simulink model "main_RI_LIEKF_GNSSOutrage"  (R2023a)
settings: Solver=FixedStepAuto  StartTime=0.0  StopTime=220  FixedStep=0.01  RelTol=1e-3
InitFcn:
  | initNavigation0612_AOA;
values from neighbouring files (symbols this model uses):
  CF_enable = 0    [initNavigation.m]
  dt = 0.01    [initNavigation.m]
  dtDelay = -0.03    [initNavigation.m]
  g0 = 9.795    [initNavigation.m]
  gam0_rad = 0/57.3    (= 0)    [initNavigation.m]
  GNSSoutragetime = 90    [initNavigation.m]
  H_sensor_type = 0    [initNavigation.m]
  KF_enable = 1    [initNavigation.m]
  P0 = diag([1*ones(3,1);0.01*ones(3,1);0.1*ones(3,1);0.001*ones(3,1);0.00001*ones(3,1)])    [initNavigation.m]
  P0_RIEKF = diag([1*ones(3,1);0.01*ones(3,1);0.1*ones(3,1);0.001*ones(3,1);0.00001*ones(3,1);      0.01*ones(3,1);[0;2;2]/57.3;[0.1;0.1;0.1]])^2    [initNavigation.m]
  pd0 = 0    [initNavigation.m]
  pe0 = 0    [initNavigation.m]
  phi0_rad = 0/57.3    (= 0)    [initNavigation.m]
  pn0 = 0    [initNavigation.m]
  psi = -178    [initNavigation.m]
  psi0_rad = 0/57.3    (= 0)    [initNavigation.m]
  state_dim = 24    [initNavigation.m]
  Time = 0:0.01:(size(traindata.AttackAngle,1) - 1)*0.01    [NNLiftCoefficientFit.m]
  vd0 = 0    [initNavigation.m]
  ve0 = 0    [initNavigation.m]
  vn0 = 0    [initNavigation.m]
undefined symbols (not defined in the file or in its folder): DiscIntNeverNeededParam, Discrete, INS_CONST, INS_EXPORT, INS_PARAM, magnitude, p, param, pInitialization, sys
libraries: simulink_extras x94, simulink x82, dspstat3 x70, sharedtransform x60, ctrlSharedLib x36, sharedTrackingLibrary x22, matrix_library x15, FMT_Model_Lib x13, deeplib x8, dspsolvers x4, vrlib x4, aerolibconvert2 x1
(part 1 of 28)
settings Model: NumberOfSteps=20  Creator=Ye Xiaoyu  LastModifiedBy=Ye Xiaoyu
settings DataIOCC: SaveFormat=Structure
settings DebuggingCC: ParameterPrecisionLossMsg=none

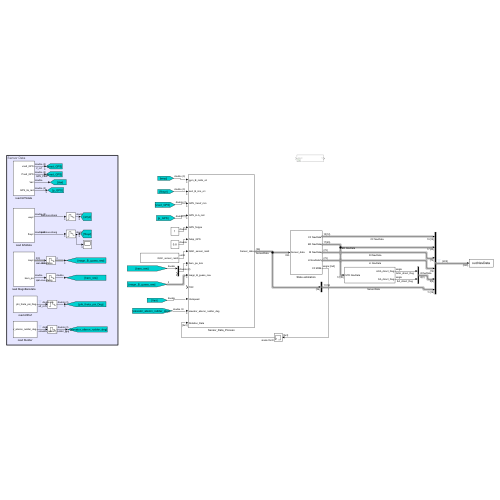
[thumbnail: Simulink's stored preview of the top-level diagram]
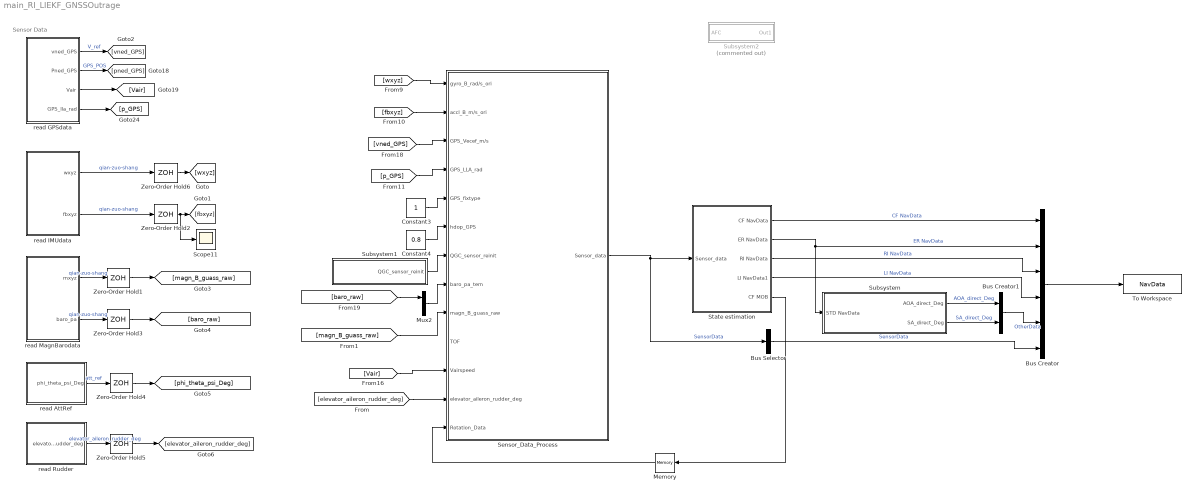
== system main_RI_LIEKF_GNSSOutrage ==
  note: Sensor Data
  Bus Creator : BusCreator  Inputs=6
  Bus Creator1 : BusCreator  Inputs=2
  Bus Selector : BusSelector  OutputSignals=BARO_Data.H_baro_TD,GPS_Data.pos_N_gps,GPS_Data.pos_E_gps,GPS_Data.pos_D_gps,GPS_Data.vn_gps,GPS_Data.ve_gps,GPS_Data.vd_gps,VairspeedData,elevator_aileron_rudder_deg,IMU_Data.gyro_B_rad/s_LPF,IMU_Data.accl_B_m/s2_LPF  OutputAsBus=on
  Constant3 : Constant
  Constant4 : Constant  Value=0.8
  Memory : Memory
  Mux2 : Mux  Inputs=2
  Scope11 : Scope
  Sensor_Data_Process : Subsystem
  State estimation : Subsystem
  Subsystem : Subsystem
  Subsystem1 : Subsystem
  Subsystem2 : Subsystem  Commented=on
  To Workspace : ToWorkspace  VariableName=NavData  SaveFormat=Timeseries  SampleTime=-1
      settings: Save2DSignal=2-D array (concatenate along first dimension)
  Zero-Order Hold{1..6} (6 alike) : ZeroOrderHold  SampleTime=dt
  read AttRef : Subsystem
  read GPSdata : Subsystem
  read IMUdata : Subsystem
  read MagnBarodata : Subsystem
  read Rudder : Subsystem
  wires:
  read GPSdata/2(Pned_GPS) -> [pned_GPS]  "GPS_POS"
  read GPSdata/1(vned_GPS) -> [vned_GPS]  "V_ref"
  read GPSdata/3(Vair) -> [Vair]
  [Vair] -> Sensor_Data_Process/11(Vairspeed)
  [baro_raw] -> Mux2/1
  Zero-Order Hold3/1 -> [baro_raw]
  Zero-Order Hold1/1 -> [magn_B_guass_raw]
  [vned_GPS] -> Sensor_Data_Process/3(GPS_Vecef_m/s)
  read MagnBarodata/2(baro_pa) -> Zero-Order Hold3/1  "qian-zuo-shang"
  Zero-Order Hold6/1 -> [wxyz]
  [p_GPS] -> Sensor_Data_Process/4(GPS_LLA_rad)
  Mux2/1 -> Sensor_Data_Process/8(baro_pa_tem)
  read MagnBarodata/1(mxyz) -> Zero-Order Hold1/1  "qian-zuo-shang"
  Constant4/1 -> Sensor_Data_Process/6(hdop_GPS)
  Constant3/1 -> Sensor_Data_Process/5(GPS_fixtype)
  [magn_B_guass_raw] -> Sensor_Data_Process/9(magn_B_guass_raw)
  [fbxyz] -> Sensor_Data_Process/2(accl_B_m/s_ori)
  Subsystem1/1(QGC_sensor_reinit) -> Sensor_Data_Process/7(QGC_sensor_reinit)
  Zero-Order Hold2/1 -> Scope11/1, [fbxyz]
  Sensor_Data_Process/1(Sensor_data) -> Bus Selector/1, State estimation/1(Sensor_data)  "SensorData"
  read GPSdata/4(GPS_lla_rad) -> [p_GPS]
  read IMUdata/1(wxyz) -> Zero-Order Hold6/1  "qian-zuo-shang"
  [wxyz] -> Sensor_Data_Process/1(gyro_B_rad/s_ori)
  read IMUdata/2(fbxyz) -> Zero-Order Hold2/1  "qian-zuo-shang"
  read AttRef/1(phi_theta_psi_Deg) -> Zero-Order Hold4/1  "att_ref"
  Zero-Order Hold4/1 -> [phi_theta_psi_Deg]
  State estimation/1(CF NavData) -> Bus Creator/1  "CF NavData"
  State estimation/2(ER NavData) -> Subsystem/1(STD NavData), Bus Creator/2  "ER NavData"
  State estimation/3(RI NavData) -> Bus Creator/3  "RI NavData"
  Bus Creator1/1 -> Bus Creator/5  "OtherData"
  Subsystem/1(AOA_direct_Deg) -> Bus Creator1/1  "AOA_direct_Deg"
  Bus Creator/1 -> To Workspace/1
  Subsystem/2(SA_direct_Deg) -> Bus Creator1/2  "SA_direct_Deg"
  Bus Selector/1 -> Bus Creator/6  "SensorData"
  read Rudder/1(elevator_aileron_rudder_deg) -> Zero-Order Hold5/1  "elevator_aileron_rudder_deg"
  Zero-Order Hold5/1 -> [elevator_aileron_rudder_deg]
  [elevator_aileron_rudder_deg] -> Sensor_Data_Process/12(elevator_aileron_rudder_deg)
  State estimation/4(LI NavData1) -> Bus Creator/4  "LI NavData"
  State estimation/5(CF MOB) -> Memory/1
  Memory/1 -> Sensor_Data_Process/13(Rotation_Data)

== system main_RI_LIEKF_GNSSOutrage/Sensor_Data_Process ==
  gyro_B_rad/s_ori : Inport
  accl_B_m/s_ori : Inport  Port=2
  GPS_Vecef_m/s : Inport  Port=3
  GPS_LLA_rad : Inport  Port=4
  GPS_fixtype : Inport  Port=5
  hdop_GPS : Inport  Port=6
  QGC_sensor_reinit : Inport  Port=7
  baro_pa_tem : Inport  Port=8
  magn_B_guass_raw : Inport  Port=9
  TOF : Inport  Port=10
  Vairspeed : Inport  Port=11
  elevator_aileron_rudder_deg : Inport  Port=12
  Rotation_Data : Inport  Port=13
  Bus Creator : BusCreator  Inputs=8
  Data Type Conversion{,1..3,5..6,8..11} (10 alike) : DataTypeConversion  OutDataTypeStr=single  SaturateOnIntegerOverflow=off  RndMeth=Floor
  Data Type Conversion4 : DataTypeConversion  OutDataTypeStr=uint8  SaturateOnIntegerOverflow=off  RndMeth=Floor
  Data Type Conversion7 : DataTypeConversion  OutDataTypeStr=double  SaturateOnIntegerOverflow=off  RndMeth=Floor
  Demux : Demux  Outputs=2
  Digital Clock : DigitalClock  SampleTime=-1
  GPS_Data_Process : Subsystem
  IMU_Data_Process : Subsystem
  Magn_Data_Process1 : Subsystem
  QGC_sensor_reinit1 : InportShadow  Port=7
  QGC_sensor_reinit2 : InportShadow  Port=7
  Subsystem : Subsystem
  TOF_Data_Process : Subsystem
  baro_Data_Process : Subsystem
  Sensor_data : Outport
  wires:
  QGC_sensor_reinit2/1 -> TOF_Data_Process/2(QGC_sensor_reinit)  "QGC_sensor_reinit"
  Data Type Conversion3/1 -> baro_Data_Process/3(baro_tem)
  Demux/2 -> Data Type Conversion3/1
  Data Type Conversion10/1 -> TOF_Data_Process/1(TOF_mm_ori)
  Data Type Conversion5/1 -> baro_Data_Process/1(baro)
  Data Type Conversion9/1 -> GPS_Data_Process/4(hdop_GPS)
  Data Type Conversion4/1 -> GPS_Data_Process/3(GPS_fixtype)
  Data Type Conversion7/1 -> GPS_Data_Process/2(GPS_LLA_rad)
  Data Type Conversion2/1 -> GPS_Data_Process/1(GPS_Vecef_m/s)
  Data Type Conversion1/1 -> IMU_Data_Process/2(accl_B_m/s_ori)
  Data Type Conversion/1 -> IMU_Data_Process/1(gyro_B_rad/s_ori)
  TOF_Data_Process/1(TOF_Data) -> Bus Creator/5
  TOF/1 -> Data Type Conversion10/1
  QGC_sensor_reinit1/1 -> Bus Creator/7  "QGC_sensor_reinit"
  hdop_GPS/1 -> Data Type Conversion9/1
  Bus Creator/1 -> Sensor_data/1
  GPS_fixtype/1 -> Data Type Conversion4/1
  GPS_Vecef_m/s/1 -> Data Type Conversion2/1
  GPS_LLA_rad/1 -> Data Type Conversion7/1
  accl_B_m/s_ori/1 -> Data Type Conversion1/1
  Magn_Data_Process1/1(MAGN_Data) -> Bus Creator/4  "MAGN_Data"
  gyro_B_rad/s_ori/1 -> Data Type Conversion/1
  baro_Data_Process/1(BARO_Data) -> Bus Creator/3  "BARO_Data"
  IMU_Data_Process/1(IMU_Data) -> Bus Creator/1  "IMU_Data"
  GPS_Data_Process/1(GPS_Data) -> Magn_Data_Process1/4(GPS), Bus Creator/2  "GPS_Data"
  QGC_sensor_reinit/1 -> GPS_Data_Process/5(QGC_sensor_reinit), baro_Data_Process/2(QGC_sensor_reinit)  "QGC_sensor_reinit"
  baro_pa_tem/1 -> Demux/1
  Demux/1 -> Data Type Conversion5/1
  Vairspeed/1 -> Data Type Conversion8/1  "VairspeedData"
  Data Type Conversion8/1 -> Subsystem/1(Vairspeed)
  Subsystem/1(VairspeedData) -> Bus Creator/6
  elevator_aileron_rudder_deg/1 -> Data Type Conversion11/1  "elevator_aileron_rudder_deg"
  Data Type Conversion11/1 -> Bus Creator/8  "elevator_aileron_rudder_deg"
  magn_B_guass_raw/1 -> Data Type Conversion6/1
  Data Type Conversion6/1 -> Magn_Data_Process1/1(magn_B_guass_ori)
  Digital Clock/1 -> Magn_Data_Process1/2(magn_B_timestep)
  Rotation_Data/1 -> Magn_Data_Process1/3(Rotation_Data)

== system main_RI_LIEKF_GNSSOutrage/State estimation ==
  Sensor_data : Inport
  0609bk : Subsystem  Commented=on
  15dim KF1 : Subsystem  Commented=on
  Bus Selector : BusSelector  OutputSignals=M_OB
  Bus_Constructor : Subsystem
  Bus_Constructor1 : Subsystem
  Bus_Constructor2 : Subsystem
  Bus_Constructor3 : Subsystem
  Constant : Constant  Value=CF_enable
  Constant1 : Constant  Value=KF_enable
  ER EKF : Subsystem
  LI EKF2 : Subsystem  Commented=on
  RI EKF_AOA_LSTM : Subsystem
  RI EKF_AOA_direct : Subsystem
  RI EKF_AOA_ref : Subsystem
  RI UKF : Subsystem  Commented=on
  bak1 : Subsystem  Commented=on
  distribute CF : Subsystem
  CF NavData : Outport
  ER NavData : Outport  Port=2
  RI NavData : Outport  Port=3
  LI NavData1 : Outport  Port=4
  CF MOB : Outport  Port=5
  wires:
  Sensor_data/1 -> ER EKF/1(Sensor_data), RI EKF_AOA_direct/1(Sensor_data), RI EKF_AOA_ref/1(Sensor_data), RI EKF_AOA_LSTM/1(Sensor_data), RI UKF/1(Sensor_data), distribute CF/1(Sensor_data)
  distribute CF/2(TranslationData) -> Bus_Constructor/2(TranlationData)
  ER EKF/1(RotationData) -> Bus_Constructor1/1(RotationData)
  ER EKF/2(TranslationData) -> Bus_Constructor1/2(TranlationData)
  ER EKF/3(INSbiasData) -> Bus_Constructor1/3(INSbiasData)
  ER EKF/4(EKFstate) -> Bus_Constructor1/4(EKFstate)
  RI EKF_AOA_LSTM/1(RotationData) -> Bus_Constructor2/1(RotationData)
  RI EKF_AOA_LSTM/2(TranslationData) -> Bus_Constructor2/2(TranlationData)
  RI EKF_AOA_LSTM/3(INSbiasData) -> Bus_Constructor2/3(INSbiasData)
  RI EKF_AOA_LSTM/4(EKF_state) -> Bus_Constructor2/4(EKFstate)
  Bus_Constructor/1(CF NavData) -> CF NavData/1
  Bus_Constructor1/1(ER EKFNav_out) -> ER NavData/1
  Bus_Constructor2/1(RI EKFNav_out) -> RI NavData/1
  RI EKF_AOA_LSTM/5(AOA/SA/Wind) -> Bus_Constructor2/5(AOA/SA/Wind)
  RI EKF_AOA_LSTM/6(GNSS enable flag) -> Bus_Constructor2/6(GNSS enable flag)
  RI EKF_AOA_direct/1(RotationData) -> Bus_Constructor3/1(RotationData)
  RI EKF_AOA_direct/2(TranslationData) -> Bus_Constructor3/2(TranlationData)
  RI EKF_AOA_direct/3(INSbiasData) -> Bus_Constructor3/3(INSbiasData)
  RI EKF_AOA_direct/4(EKF_state) -> Bus_Constructor3/4(EKFstate)
  RI EKF_AOA_direct/5(AOA/SA/Wind) -> Bus_Constructor3/5(AOA/SA/Wind)
  RI EKF_AOA_direct/6(GNSS enable flag) -> Bus_Constructor3/6(GNSS enable flag)
  Bus_Constructor3/1(RI EKFNav_out) -> LI NavData1/1
  distribute CF/1(RotationData) -> Bus Selector/1, Bus_Constructor/1(RotationData)
  Bus Selector/1 -> CF MOB/1  "<M_OB>"

== system main_RI_LIEKF_GNSSOutrage/Subsystem ==
  STD NavData : Inport
  Bus Selector : BusSelector  OutputSignals=RotationData.theta_rad,TranlationData.vn_m/s,TranlationData.ve_m/s,TranlationData.vd_m/s,RotationData.psi_rad
  Constant : Constant  Value=0
  Data Type Conversion : DataTypeConversion  OutDataTypeStr=single  SaturateOnIntegerOverflow=off  RndMeth=Floor
  Data Type Conversion1 : DataTypeConversion  OutDataTypeStr=single  SaturateOnIntegerOverflow=off  RndMeth=Floor
  MATLAB Function : MATLAB Function  TreatAsAtomicUnit=on
  Mux : Mux  Inputs=3
  Subsystem1 : Subsystem
  Subsystem3 : Subsystem
  Switch : Switch  Threshold=1  SaturateOnIntegerOverflow=off  InputSameDT=off
  Switch1 : Switch  Threshold=1  SaturateOnIntegerOverflow=off  InputSameDT=off
  AOA_direct_Deg : Outport
  SA_direct_Deg : Outport  Port=2
  wires:
  Bus Selector/2 -> Mux/1  "<vn_m/s>"
  Bus Selector/3 -> Mux/2  "<ve_m/s>"
  STD NavData/1 -> Bus Selector/1
  Bus Selector/4 -> Mux/3  "<vd_m/s>"
  Bus Selector/1 -> Subsystem3/1(RIEKF_att_Deg)  "<theta_rad>"
  Subsystem3/1(AOA_direct_Deg) -> Switch/1
  Mux/1 -> Subsystem1/1(vel_NED), Subsystem3/2(vel_NED)
  Data Type Conversion/1 -> AOA_direct_Deg/1
  Bus Selector/5 -> Subsystem3/3(psi_Deg)  "<psi_rad>"
  Constant/1 -> Switch1/3, Switch/3
  Subsystem1/1(AOA_Estimation_flag) -> Switch1/2, Switch/2, Subsystem3/Enable
  Switch/1 -> Data Type Conversion/1  "INSstate_Rab"
  Subsystem3/2(SA_direct_Deg) -> MATLAB Function/1(dpsi)
  Data Type Conversion1/1 -> SA_direct_Deg/1
  Switch1/1 -> Data Type Conversion1/1  "INSstate_Rab"
  MATLAB Function/1(y) -> Switch1/1

== system main_RI_LIEKF_GNSSOutrage/Subsystem1 ==
  Compare To Constant : simulink/Logic and Bit Operations/Compare To Constant  relop=<=  const=2.1  OutDataTypeStr=boolean
  Compare To Constant1 : simulink/Logic and Bit Operations/Compare To Constant  relop=>=  const=2  OutDataTypeStr=boolean
  Constant5 : Constant  OutDataTypeStr=uint8
  Constant8 : Constant  Value=0  OutDataTypeStr=uint8
  Digital Clock : DigitalClock  SampleTime=dt
  Logical Operator1 : Logic  AllPortsSameDT=off  OutDataTypeStr=boolean
  Switch3 : Switch  Criteria=u2 > Threshold  SaturateOnIntegerOverflow=off  InputSameDT=off
  QGC_sensor_reinit : Outport
  wires:
  Digital Clock/1 -> Compare To Constant1/1, Compare To Constant/1
  Logical Operator1/1 -> Switch3/2
  Constant5/1 -> Switch3/1
  Compare To Constant1/1 -> Logical Operator1/1
  Compare To Constant/1 -> Logical Operator1/2
  Constant8/1 -> Switch3/3
  Switch3/1 -> QGC_sensor_reinit/1

== system main_RI_LIEKF_GNSSOutrage/Subsystem2 ==
  AFC : Inport
  Data Type Conversion18 : DataTypeConversion  OutDataTypeStr=single  SaturateOnIntegerOverflow=off  RndMeth=Floor
  Demux : Demux  Outputs=3
  MATLAB Function1 : MATLAB Function  TreatAsAtomicUnit=on
  Mux2 : Mux  Inputs=2
  Mux29 : Mux  Inputs=2
  Out1 : Outport
  wires:
  Mux2/1 -> Mux29/1
  Data Type Conversion18/1 -> Mux29/2  "AFC"
  Demux/2 -> Mux2/2
  Demux/1 -> Mux2/1
  Demux/3 -> MATLAB Function1/1(x)
  Mux29/1 -> Out1/1
  MATLAB Function1/1(angleHeadingAB0to360) -> Data Type Conversion18/1
  AFC/1 -> Demux/1

== system main_RI_LIEKF_GNSSOutrage/read AttRef ==
  From Workspace : FromWorkspace  VariableName=[All.t',All.thetaL]
  From Workspace1 : FromWorkspace  VariableName=[All.t',All.phiL]
  From Workspace2 : FromWorkspace  VariableName=[All.t',All.psiL]
  Mux3 : Mux  Inputs=3
  phi_theta_psi_Deg : Outport
  wires:
  Mux3/1 -> phi_theta_psi_Deg/1
  From Workspace/1 -> Mux3/2
  From Workspace1/1 -> Mux3/1
  From Workspace2/1 -> Mux3/3

== system main_RI_LIEKF_GNSSOutrage/read GPSdata ==
  Add1 : Sum
  Add2 : Sum
  Constant1 : Constant  Value=1.7
  Constant2 : Constant  Value=0.5311
  Degrees to Radians : simulink_extras/Transformations/Degrees to Radians
  Degrees to Radians1 : simulink_extras/Transformations/Degrees to Radians
  From Workspace : FromWorkspace  VariableName=[All.t',All.ve]
  From Workspace1 : FromWorkspace  VariableName=[All.t',All.vn]
  From Workspace2 : FromWorkspace  VariableName=[All.t',All.mhdot]
  From Workspace3 : FromWorkspace  VariableName=[All.t',All.Yeast]
  From Workspace4 : FromWorkspace  VariableName=[All.t',All.Xnorth]
  From Workspace5 : FromWorkspace  VariableName=[All.t',All.mh]
  From Workspace6 : FromWorkspace  VariableName=[All.t',All.Vc]
  From Workspace7 : FromWorkspace  VariableName=[All.t',All.lat]
  From Workspace8 : FromWorkspace  VariableName=[All.t',All.lon]
  From Workspace9 : FromWorkspace  VariableName=[All.t',All.mh]
  Gain : Gain  Gain=1/3.6
  Gain1 : Gain  Gain=-1
  Gain2 : Gain  Gain=-1
  Gain3 : Gain  Gain=1.0626
  Mux : Mux  Inputs=3
  Mux1 : Mux  Inputs=3
  Mux2 : Mux  Inputs=3
  Scope{,1..2,4} (4 alike) : Scope
  vned_GPS : Outport
  Pned_GPS : Outport  Port=2
  Vair : Outport  Port=3
  GPS_lla_rad : Outport  Port=4
  wires:
  From Workspace2/1 -> Gain1/1
  From Workspace5/1 -> Gain2/1
  From Workspace/1 -> Mux/2  "ve"
  From Workspace1/1 -> Mux/1  "vn"
  From Workspace6/1 -> Gain/1
  From Workspace4/1 -> Mux1/1
  From Workspace3/1 -> Mux1/2
  Gain1/1 -> Mux/3
  Gain2/1 -> Mux1/3
  From Workspace9/1 -> Mux2/3  "altitude"
  Mux2/1 -> Scope/1, GPS_lla_rad/1
  From Workspace8/1 -> Degrees to Radians1/1  "lon"
  From Workspace7/1 -> Degrees to Radians/1  "lat"
  Degrees to Radians/1 -> Mux2/1
  Degrees to Radians1/1 -> Mux2/2
  Mux1/1 -> Pned_GPS/1, Scope1/1
  Mux/1 -> vned_GPS/1, Scope2/1
  Add1/1 -> ?
  Constant1/1 -> Add1/2
  ? -> Scope4/1
  ? -> Add1/1
  Gain/1 -> Gain3/1
  Gain3/1 -> Add2/1
  Constant2/1 -> Add2/2
  Add2/1 -> Vair/1

== system main_RI_LIEKF_GNSSOutrage/read IMUdata ==
  Bus Creator : BusCreator  Inputs=3
  Bus Creator1 : BusCreator  Inputs=3
  Degrees to Radians : simulink_extras/Transformations/Degrees to Radians
  From Workspace : FromWorkspace  VariableName=[All.t',All.q]
  From Workspace1 : FromWorkspace  VariableName=[All.t',All.p]
  From Workspace2 : FromWorkspace  VariableName=[All.t',All.r]
  From Workspace3 : FromWorkspace  VariableName=[All.t',All.Nx]
  From Workspace4 : FromWorkspace  VariableName=[All.t',All.Ny]
  From Workspace5 : FromWorkspace  VariableName=[All.t',All.Nz]
  Gain1 : Gain  Gain=-1
  Gain2 : Gain  Gain=9.81
  Scope : Scope
  Scope1 : Scope
  Scope2 : Scope
  wxyz : Outport
  fbxyz : Outport  Port=2
  wires:
  Bus Creator1/1 -> Scope1/1, Gain2/1
  Bus Creator/1 -> Degrees to Radians/1, Scope/1
  Gain2/1 -> fbxyz/1
  From Workspace2/1 -> Bus Creator/3
  From Workspace5/1 -> Gain1/1
  From Workspace3/1 -> Bus Creator1/1
  From Workspace4/1 -> Bus Creator1/2
  Gain1/1 -> Bus Creator1/3
  From Workspace1/1 -> Bus Creator/1
  From Workspace/1 -> Bus Creator/2
  Degrees to Radians/1 -> Scope2/1, wxyz/1

== system main_RI_LIEKF_GNSSOutrage/read MagnBarodata ==
  Bus Creator : BusCreator  Inputs=3
  From Workspace1 : FromWorkspace  VariableName=[All.t',All.mx]
  From Workspace2 : FromWorkspace  VariableName=[All.t',All.my]
  From Workspace3 : FromWorkspace  VariableName=[All.t',All.baro]
  From Workspace6 : FromWorkspace  VariableName=[All.t',All.mz]
  Gain1 : Gain  Gain=-1
  Scope : Scope
  Scope1 : Scope
  mxyz : Outport
  baro_pa : Outport  Port=2
  wires:
  From Workspace2/1 -> Bus Creator/2
  From Workspace1/1 -> Bus Creator/1
  Bus Creator/1 -> mxyz/1, Scope/1
  From Workspace3/1 -> baro_pa/1
  From Workspace6/1 -> Gain1/1
  Gain1/1 -> Bus Creator/3

== system main_RI_LIEKF_GNSSOutrage/read Rudder ==
  From Workspace : FromWorkspace  VariableName=[All.t',All.dacl]
  From Workspace1 : FromWorkspace  VariableName=[All.t',All.decl]
  From Workspace2 : FromWorkspace  VariableName=[All.t',All.drcl]
  Mux3 : Mux  Inputs=3
  elevator_aileron_rudder_deg : Outport
  wires:
  Mux3/1 -> elevator_aileron_rudder_deg/1
  From Workspace/1 -> Mux3/2
  From Workspace1/1 -> Mux3/1
  From Workspace2/1 -> Mux3/3

== system main_RI_LIEKF_GNSSOutrage/Sensor_Data_Process/GPS_Data_Process ==
  note: GPS_fixtype:
      | 0: 定位不可用或无效
      | 1:单点定位
      | 2:伪距差分
      | 4:RTK固定解
  GPS_Vecef_m/s : Inport
  GPS_LLA_rad : Inport  Port=2
  GPS_fixtype : Inport  Port=3
  hdop_GPS : Inport  Port=4
  QGC_sensor_reinit : Inport  Port=5
  Bus Creator : BusCreator  Inputs=13
  Demux : Demux  Outputs=3
  Demux1 : Demux  Outputs=3
  Demux3 : Demux  Outputs=3
  GPS_fixtype1 : InportShadow  Port=3
  LLA2NED : Subsystem
  heading_GPS : Subsystem
  GPS_Data : Outport
  wires:
  hdop_GPS/1 -> Bus Creator/13  "hdop_GPS"
  heading_GPS/2(heading_GPS_valid) -> Bus Creator/11  "heading_GPS_valid"
  heading_GPS/1(heading_GPS_rad) -> Bus Creator/10  "heading_GPS_rad"
  LLA2NED/2(gpsvNEDout) -> Demux/1
  GPS_Vecef_m/s/1 -> LLA2NED/3(GPS_Vecef_m/s)
  Demux1/3 -> Bus Creator/6  "pos_D_gps"
  Demux1/2 -> Bus Creator/5  "pos_E_gps"
  Demux1/1 -> Bus Creator/4  "pos_N_gps"
  QGC_sensor_reinit/1 -> LLA2NED/4(QGC_sensor_reinit)  "QGC_sensor_reinit"
  GPS_fixtype/1 -> Bus Creator/12  "fixtype_gps"
  Demux3/1 -> Bus Creator/1  "lat_gps"
  Demux3/2 -> Bus Creator/2  "lon_gps"
  Demux/2 -> Bus Creator/8  "ve_gps"
  GPS_LLA_rad/1 -> LLA2NED/1(gps_LLA_rad), Demux3/1
  Demux/1 -> Bus Creator/7  "vn_gps"
  Demux/3 -> Bus Creator/9  "vd_gps"
  Demux3/3 -> Bus Creator/3  "H_gps"
  Bus Creator/1 -> GPS_Data/1
  GPS_fixtype1/1 -> LLA2NED/2(GPSfixtype)  "fixtype_gps"
  LLA2NED/1("gpsposNEDout ") -> Demux1/1, heading_GPS/1(Vned)

== system main_RI_LIEKF_GNSSOutrage/Sensor_Data_Process/IMU_Data_Process ==
  gyro_B_rad/s_ori : Inport
  accl_B_m/s_ori : Inport  Port=2
  Bias Eliminate : Subsystem
  Bus Creator : BusCreator  Inputs=2
  accl_preprocessing2 : Subsystem  Commented=on
  gyro_preprocessing2 : Subsystem  Commented=on
  IMU_Data : Outport  PortDimensions=6
  wires:
  gyro_B_rad/s_ori/1 -> Bias Eliminate/1(gyro_B_rad/s_ori)  "gyro_B_rad/s_LPF"
  Bias Eliminate/1(Out1) -> Bus Creator/1  "gyro_B_rad/s_LPF"
  accl_B_m/s_ori/1 -> Bus Creator/2  "accl_B_m/s2_LPF"
  Bus Creator/1 -> IMU_Data/1

== system main_RI_LIEKF_GNSSOutrage/Sensor_Data_Process/Magn_Data_Process1 ==
  magn_B_guass_ori : Inport
  magn_B_timestep : Inport  Port=2
  Rotation_Data : Inport  Port=3
  GPS : Inport  Port=4
  Bus Creator : BusCreator  Inputs=2
  Gauss_to_uT : Gain  Gain=100
  Mag_Data_Process : Subsystem
  Scope : Scope
  Sensor_Valid : Subsystem  mask{mag_min=-30000, mag_max=30000, timeout=1000}
      mask prompts: mag_min "Mag min (gauss)"; mag_max "Mag max (gauss)"; timeout "Timeout (ms)"
  Zero-Order Hold : ZeroOrderHold  SampleTime=-1
  MAGN_Data : Outport
  wires:
  magn_B_guass_ori/1 -> Gauss_to_uT/1, Sensor_Valid/1(mag_B_gauss)
  magn_B_timestep/1 -> Sensor_Valid/2(timestamp_ms)
  Gauss_to_uT/1 -> Mag_Data_Process/1(mag_B_uT)
  Sensor_Valid/1(valid) -> Scope/1, Mag_Data_Process/2(mag_valid)
  Rotation_Data/1 -> Mag_Data_Process/3(DCM_OB)
  GPS/1 -> Mag_Data_Process/4(GPS_Data)
  Bus Creator/1 -> MAGN_Data/1
  Mag_Data_Process/1(mag_normalized_B) -> Zero-Order Hold/1  "mag_norm_B"
  Mag_Data_Process/2(mag_quality) -> Bus Creator/2  "mag_quality"
  Zero-Order Hold/1 -> Bus Creator/1  "mag_norm_B"

== system main_RI_LIEKF_GNSSOutrage/Sensor_Data_Process/Subsystem ==
  Vairspeed : Inport
  Constant : Constant  Value=0  OutDataTypeStr=single
  Mux : Mux  Inputs=3
  TD_baro : Subsystem
  Terminator : Terminator
  VairspeedData : Outport
  wires:
  TD_baro/2(H_baro_TD) -> Mux/1
  Constant/1 -> Mux/3, Mux/2
  Mux/1 -> VairspeedData/1  "VairspeedData"
  Vairspeed/1 -> TD_baro/1(H_baro)
  TD_baro/1(vH_baro_TD) -> Terminator/1  "vH_baro_m/s_TD"

== system main_RI_LIEKF_GNSSOutrage/Sensor_Data_Process/TOF_Data_Process ==
  TOF_mm_ori : Inport
  QGC_sensor_reinit : Inport  Port=2
  Bus Creator1 : BusCreator  Inputs=4
  Data Type Conversion : DataTypeConversion  OutDataTypeStr=uint8  SaturateOnIntegerOverflow=off  RndMeth=Floor
  Data Type Conversion1 : DataTypeConversion  OutDataTypeStr=single  SaturateOnIntegerOverflow=off  RndMeth=Floor
  Demux : Demux  Outputs=3
  Gain : Gain  Gain=0.01
  Scope : Scope  NumInputPorts=2
  Scope1 : Scope  NumInputPorts=2
  Sum : Sum  Inputs=|-+
  TD_baro : Subsystem
  reinit_TOF : Subsystem
  TOF_Data : Outport
  wires:
  Sum/1 -> Data Type Conversion1/1, Scope1/2  "TOF_Dist_m"
  reinit_TOF/1(dataout) -> Sum/1, Scope1/1
  QGC_sensor_reinit/1 -> reinit_TOF/1(QGC_sensor_reinit)
  Data Type Conversion/1 -> Bus Creator1/4  "TOF_sts"
  Gain/1 -> reinit_TOF/2(Data), Sum/2  "TOF_Dist_m"
  TD_baro/1(vH_TOF_TD) -> Bus Creator1/1, Scope/1  "vH_TOF_m/s_TD"
  Bus Creator1/1 -> TOF_Data/1  "TOF_Data"
  Demux/2 -> Bus Creator1/3  "TOF_Inten"
  TOF_mm_ori/1 -> Demux/1
  Demux/1 -> Gain/1
  Demux/3 -> Data Type Conversion/1  "TOF_sts"
  TD_baro/2(H_TOF_TD) -> Scope/2, Bus Creator1/2  "H_TOF_TD"
  Data Type Conversion1/1 -> TD_baro/1(H_TOF)  "补偿姿态前"

== system main_RI_LIEKF_GNSSOutrage/Sensor_Data_Process/baro_Data_Process ==
  baro : Inport
  QGC_sensor_reinit : Inport  Port=2
  baro_tem : Inport  Port=3
  Add : Sum
  Bus Creator : BusCreator  Inputs=2
  Constant : Constant  Value=0  OutDataTypeStr=single
  Constant1 : Constant  Value=-0.2704  OutDataTypeStr=single
  From Workspace : FromWorkspace  Commented=on  VariableName=[All.t',All.Alt_Ps]
  Gain : Gain  Gain=0.01
  Gain1 : Gain  Gain=1.0530
  Pressure2Height : Subsystem
  Scope : Scope
  Scope1 : Scope  Commented=on  NumInputPorts=2
  Sum : Sum  Inputs=|+-
  Sum1 : Sum  Commented=on  Inputs=|+-
  Sum2 : Sum  Inputs=|+-
  Switch : Switch  Criteria=u2 > Threshold  Threshold=31  SaturateOnIntegerOverflow=off  InputSameDT=off
  TD_baro : Subsystem
  TemCompensate1 : Subsystem
  To Workspace : ToWorkspace  VariableName=H_baro_TD  SaveFormat=Timeseries  SampleTime=-1
  reinit_baro0 : Subsystem
  reinit_baro1 : Subsystem  Commented=on
  BARO_Data : Outport  PortDimensions=2
  wires:
  baro_tem/1 -> TemCompensate1/1(baro_tem), Switch/2  "AFCbarotem"
  Add/1 -> TD_baro/1(H_baro)  "AFC4"
  Switch/1 -> Sum2/2
  baro/1 -> Gain/1  "AFC4"
  Constant/1 -> Switch/1
  TemCompensate1/1(bias) -> Switch/3
  Sum2/1 -> Sum/1, reinit_baro0/2(Data)
  TD_baro/2(H_baro_TD) -> Sum2/1  "H_baro_TD"
  Sum/1 -> Scope1/2, Scope/1, To Workspace/1, Bus Creator/2  "H_baro_TD"
  reinit_baro0/1(dataout) -> Sum/2
  QGC_sensor_reinit/1 -> reinit_baro1/1(QGC_sensor_reinit), reinit_baro0/1(QGC_sensor_reinit)
  Bus Creator/1 -> BARO_Data/1
  Gain/1 -> Pressure2Height/1(baro)
  TD_baro/1(vH_baro_TD) -> Bus Creator/1  "vH_baro_m/s_TD"
  From Workspace/1 -> reinit_baro1/2(Data), Sum1/1
  reinit_baro1/1(dataout) -> Sum1/2
  Sum1/1 -> Scope1/1
  Pressure2Height/1(H_baro) -> Gain1/1  "AFC4"
  Gain1/1 -> Add/1  "AFC4"
  Constant1/1 -> Add/2

== system main_RI_LIEKF_GNSSOutrage/State estimation/0609bk ==
  Sensor_data : Inport
  Bus_Constructor : Subsystem
  Data Store Memory : DataStoreMemory  DataStoreName=feedback_flag_18dim  WriteAfterWriteMsg=warning  ShowAdditionalParam=off
  Data Store Memory1 : DataStoreMemory  DataStoreName=GPS_enable  WriteAfterWriteMsg=warning  ShowAdditionalParam=off
  Data Store Read : DataStoreRead  DataStoreName=GPS_enable  IndexOptions=Index vector (dialog)  Indices=1  OutputSizes=1
  Error State Kalman Filter : Subsystem
  INS propogation : Subsystem
  Sensor_data1 : InportShadow
  TranslationData : Outport
  RotationData : Outport  Port=2
  delta_state : Outport  Port=3
  wires:
  Sensor_data1/1 -> Error State Kalman Filter/1(Sensor_data)
  Bus_Constructor/2(RotationData) -> RotationData/1
  Bus_Constructor/1(TranslationData) -> TranslationData/1
  INS propogation/1(INSstate) -> Bus_Constructor/1(INSstate), Error State Kalman Filter/2(INS state)
  Sensor_data/1 -> INS propogation/1(Sensor_data)
  Error State Kalman Filter/1(state) -> INS propogation/2(state)

== system main_RI_LIEKF_GNSSOutrage/State estimation/15dim KF1 ==
  Sensor_data : Inport
  Bus_Constructor : Subsystem
  Data Store Memory : DataStoreMemory  DataStoreName=feedback_flag  WriteAfterWriteMsg=warning  ShowAdditionalParam=off
  Error State Kalman Filter : Subsystem
  INS propogation : Subsystem
  Scope : Scope
  Sensor_data1 : InportShadow
  Subsystem2 : Subsystem  Commented=on
      settings: PortSchema="{\"entries\":[{\"content\":{\"sides\":[{\"content\":{\"connectorIds\":[\"In1\",\"In2\",\"In3\",\"In4\",\"In5\",\"In6\",\"In7\"]},\"type\":\"ConnectorPlacement.EquallySpacedRectSide\",\"uuid\":\"d8a1abfc-3a64-4957-9a04-f862f8438181\"},{\"content\":{\"connectorIds\":[\"Out1\",\"Out2\"],\"side\":\"RIGHT\"},\"type\":\"ConnectorPlacement.EquallySpacedRectSide\",\"uuid\":\"ef8725ce-d750-4a63-8901-4156c775c830\"},{\"content\":{\"connectorIds\":[\"In8\"],\"side\":\"TOP\"},\"type\":\"ConnectorPlacement.EquallySpacedRectSide\",\"uuid\":\"854b71eb-e012-4efc-86b0-6708fad9ae5c\"},{\"content\":{\"connectorIds\":[],\"side\":\"BOTTOM\"},\"type\":\"ConnectorPlacement.EquallySpacedRectSide\",\"uuid\":\"0d7ed0fe-5852-4514-b91b-1c224e1f49d3\"}]},\"type\":\"ConnectorPlacement.EquallySpacedConnector\",\"uuid\":\"3a6989db-34d3-4b77-867e-5841d7913155\"}],\"packageUris\":[\"http://schema.mathworks.com/mf0/Connector/R2020b\"],\"version\":\"1.0\"}"
  TranslationData : Outport
  RotationData : Outport  Port=2
  wires:
  Sensor_data1/1 -> Error State Kalman Filter/1(Sensor_data)
  Error State Kalman Filter/3(covariance) -> Scope/1
  Bus_Constructor/2(RotationData) -> RotationData/1
  Bus_Constructor/1(TranslationData) -> TranslationData/1
  INS propogation/1(INSstate) -> Bus_Constructor/1(INSstate), Error State Kalman Filter/2(INS state)
  Error State Kalman Filter/2(Measuemrnt Enable Flag) -> INS propogation/2(Measuemrnt Enable Flag)
  Error State Kalman Filter/1(delta_state) -> INS propogation/3(delta_state)
  Sensor_data/1 -> INS propogation/1(Sensor_data)

== system main_RI_LIEKF_GNSSOutrage/State estimation/Bus_Constructor ==
  RotationData : Inport
  TranlationData : Inport  Port=2
  Bus Creator : BusCreator  Inputs=3
  Bus Creator1 : BusCreator  Inputs=3
  Bus Selector : BusSelector  OutputSignals=phi_rad,theta_rad,psi_rad,bias_g
  Data Type Conversion1 : DataTypeConversion  OutDataTypeStr=single  SaturateOnIntegerOverflow=off  RndMeth=Floor
  Radians to Degrees1 : simulink_extras/Transformations/Radians to Degrees
  Radians to Degrees2 : simulink_extras/Transformations/Radians to Degrees
  Radians to Degrees3 : simulink_extras/Transformations/Radians to Degrees
  CF NavData : Outport
  wires:
  RotationData/1 -> Bus Selector/1
  Bus Creator/1 -> CF NavData/1
  TranlationData/1 -> Bus Creator/1  "TranlationData"
  Bus Selector/1 -> Radians to Degrees3/1  "<phi_rad>"
  Bus Creator1/1 -> Bus Creator/2  "RotationData"
  Bus Selector/2 -> Radians to Degrees2/1  "<theta_rad>"
  Bus Selector/3 -> Radians to Degrees1/1  "<psi_rad>"
  Radians to Degrees1/1 -> Bus Creator1/1  "phi_rad"
  Radians to Degrees2/1 -> Bus Creator1/2  "theta_rad"
  Radians to Degrees3/1 -> Bus Creator1/3  "psi_rad"
  Bus Selector/4 -> Bus Creator/3  "<bias_g>"

== system main_RI_LIEKF_GNSSOutrage/State estimation/Bus_Constructor1 ==
  RotationData : Inport
  TranlationData : Inport  Port=2
  INSbiasData : Inport  Port=3
  EKFstate : Inport  Port=4
  Bus Creator : BusCreator  Inputs=4
  Rotation_output : Subsystem
  ER EKFNav_out : Outport
  wires:
  RotationData/1 -> Rotation_output/1(RotationData)  "RotationData"
  Bus Creator/1 -> ER EKFNav_out/1
  TranlationData/1 -> Bus Creator/1  "TranlationData"
  Rotation_output/1(psi_theta_phi_rad) -> Bus Creator/2  "RotationData"
  INSbiasData/1 -> Bus Creator/3  "INSbiasData"
  EKFstate/1 -> Bus Creator/4  "EKFstate"

== system main_RI_LIEKF_GNSSOutrage/State estimation/Bus_Constructor2 ==
  RotationData : Inport
  TranlationData : Inport  Port=2
  INSbiasData : Inport  Port=3
  EKFstate : Inport  Port=4
  AOA/SA/Wind : Inport  Port=5
  GNSS enable flag : Inport  Port=6
  Bus Creator : BusCreator  Inputs=6
  Rotation_output : Subsystem
  RI EKFNav_out : Outport
  wires:
  EKFstate/1 -> Bus Creator/4  "EKFstate"
  INSbiasData/1 -> Bus Creator/3  "INSbiasData"
  Rotation_output/1(psi_theta_phi_rad) -> Bus Creator/2  "RotationData"
  TranlationData/1 -> Bus Creator/1  "TranlationData"
  Bus Creator/1 -> RI EKFNav_out/1
  RotationData/1 -> Rotation_output/1(RotationData)  "RotationData"
  AOA/SA/Wind/1 -> Bus Creator/5  "AOA/SA/Wind"
  GNSS enable flag/1 -> Bus Creator/6  "GNSS enable flag"

== system main_RI_LIEKF_GNSSOutrage/State estimation/Bus_Constructor3 ==
  RotationData : Inport
  TranlationData : Inport  Port=2
  INSbiasData : Inport  Port=3
  EKFstate : Inport  Port=4
  AOA/SA/Wind : Inport  Port=5
  GNSS enable flag : Inport  Port=6
  Bus Creator : BusCreator  Inputs=6
  Rotation_output : Subsystem
  RI EKFNav_out : Outport
  wires:
  GNSS enable flag/1 -> Bus Creator/6  "GNSS enable flag"
  AOA/SA/Wind/1 -> Bus Creator/5  "AOA/SA/Wind"
  RotationData/1 -> Rotation_output/1(RotationData)  "RotationData"
  Bus Creator/1 -> RI EKFNav_out/1
  TranlationData/1 -> Bus Creator/1  "TranlationData"
  Rotation_output/1(psi_theta_phi_rad) -> Bus Creator/2  "RotationData"
  INSbiasData/1 -> Bus Creator/3  "INSbiasData"
  EKFstate/1 -> Bus Creator/4  "EKFstate"

== system main_RI_LIEKF_GNSSOutrage/State estimation/ER EKF ==
  Sensor_data : Inport
  Bus_Constructor : Subsystem
  Data Store Memory : DataStoreMemory  DataStoreName=feedback_flag_18dim  WriteAfterWriteMsg=warning  ShowAdditionalParam=off
  Data Store Memory1 : DataStoreMemory  DataStoreName=GPS_enable  WriteAfterWriteMsg=warning  ShowAdditionalParam=off
  Data Store Read : DataStoreRead  DataStoreName=GPS_enable  IndexOptions=Index vector (dialog)  Indices=1  OutputSizes=1
  Error State Kalman Filter : Subsystem
  INS propogation : Subsystem
  Sensor_data1 : InportShadow
  RotationData : Outport
  TranslationData : Outport  Port=2
  INSbiasData : Outport  Port=3
  EKFstate : Outport  Port=4
  wires:
  Sensor_data/1 -> INS propogation/1(Sensor_data)
  Error State Kalman Filter/1(delta_state) -> INS propogation/3(delta_state)
  Error State Kalman Filter/2(Measuemrnt Enable Flag) -> INS propogation/2(Measuemrnt Enable Flag)
  INS propogation/1(INSstate) -> Bus_Constructor/1(INSstate), Error State Kalman Filter/2(INS state)
  Bus_Constructor/1(TranslationData) -> TranslationData/1
  Bus_Constructor/2(RotationData) -> RotationData/1
  Sensor_data1/1 -> Error State Kalman Filter/1(Sensor_data)
  Bus_Constructor/3(INSbiasData) -> INSbiasData/1
  Error State Kalman Filter/3(EKFState) -> EKFstate/1

== system main_RI_LIEKF_GNSSOutrage/State estimation/LI EKF2 ==
  Sensor_data : Inport
  Bus_Constructor : Subsystem
  Data Store Memory : DataStoreMemory  DataStoreName=feedback_flag_18dim_LIEKF  WriteAfterWriteMsg=warning  ShowAdditionalParam=off
  Data Store Memory1 : DataStoreMemory  DataStoreName=GPS_enable_LIEKF  WriteAfterWriteMsg=warning  ShowAdditionalParam=off
  Error State Kalman Filter : Subsystem
  INS propogation : Subsystem
  Sensor_data1 : InportShadow
  RotationData : Outport
  TranslationData : Outport  Port=2
  INSbiasData : Outport  Port=3
  EKF_state : Outport  Port=4
  AOA/SA/Wind : Outport  Port=5
  GNSS enable flag : Outport  Port=6
  wires:
  Sensor_data1/1 -> Error State Kalman Filter/1(Sensor_data)
  Bus_Constructor/2(RotationData) -> RotationData/1
  Bus_Constructor/1(TranslationData) -> TranslationData/1
  INS propogation/1(INSstate) -> Error State Kalman Filter/2(INS state), Bus_Constructor/1(INSstate)
  Error State Kalman Filter/2(Measuemrnt Enable Flag) -> INS propogation/2(Measuemrnt Enable Flag)
  Error State Kalman Filter/1(delta_state) -> INS propogation/3(delta_state)
  Sensor_data/1 -> INS propogation/1(Sensor_data)
  Error State Kalman Filter/3(EKFstate) -> EKF_state/1
  Bus_Constructor/3(INSbiasData) -> INSbiasData/1
  Bus_Constructor/4(AOA/SA/Wind) -> AOA/SA/Wind/1
  Bus_Constructor/5(GNSS enable flag) -> GNSS enable flag/1

== system main_RI_LIEKF_GNSSOutrage/State estimation/RI EKF_AOA_LSTM ==
  Sensor_data : Inport
  Bus_Constructor : Subsystem
  Data Store Memory : DataStoreMemory  DataStoreName=feedback_flag_18dim_RIEKF  WriteAfterWriteMsg=warning  ShowAdditionalParam=off
  Data Store Memory1 : DataStoreMemory  DataStoreName=GPS_enable_RIEKF  WriteAfterWriteMsg=warning  ShowAdditionalParam=off
  Error State Kalman Filter : Subsystem
  INS propogation : Subsystem
  Sensor_data1 : InportShadow
  RotationData : Outport
  TranslationData : Outport  Port=2
  INSbiasData : Outport  Port=3
  EKF_state : Outport  Port=4
  AOA/SA/Wind : Outport  Port=5
  GNSS enable flag : Outport  Port=6
  wires:
  Sensor_data1/1 -> Error State Kalman Filter/1(Sensor_data)
  Bus_Constructor/2(RotationData) -> RotationData/1
  Bus_Constructor/1(TranslationData) -> TranslationData/1
  INS propogation/1(INSstate) -> Error State Kalman Filter/2(INS state), Bus_Constructor/1(INSstate)
  Error State Kalman Filter/2(Measuemrnt Enable Flag) -> INS propogation/2(Measuemrnt Enable Flag)
  Error State Kalman Filter/1(delta_state) -> INS propogation/3(delta_state)
  Sensor_data/1 -> INS propogation/1(Sensor_data)
  Error State Kalman Filter/3(EKFstate) -> EKF_state/1
  Bus_Constructor/3(INSbiasData) -> INSbiasData/1
  Bus_Constructor/4(AOA/SA/Wind) -> AOA/SA/Wind/1
  Bus_Constructor/5(GNSS enable flag) -> GNSS enable flag/1

== system main_RI_LIEKF_GNSSOutrage/State estimation/RI EKF_AOA_direct ==
  Sensor_data : Inport
  Bus_Constructor : Subsystem
  Data Store Memory : DataStoreMemory  DataStoreName=feedback_flag_18dim_RIEKF  WriteAfterWriteMsg=warning  ShowAdditionalParam=off
  Data Store Memory1 : DataStoreMemory  DataStoreName=GPS_enable_RIEKF  WriteAfterWriteMsg=warning  ShowAdditionalParam=off
  Error State Kalman Filter : Subsystem
  INS propogation : Subsystem
  Sensor_data1 : InportShadow
  RotationData : Outport
  TranslationData : Outport  Port=2
  INSbiasData : Outport  Port=3
  EKF_state : Outport  Port=4
  AOA/SA/Wind : Outport  Port=5
  GNSS enable flag : Outport  Port=6
  wires:
  Bus_Constructor/5(GNSS enable flag) -> GNSS enable flag/1
  Bus_Constructor/4(AOA/SA/Wind) -> AOA/SA/Wind/1
  Bus_Constructor/3(INSbiasData) -> INSbiasData/1
  Error State Kalman Filter/3(EKFstate) -> EKF_state/1
  Sensor_data/1 -> INS propogation/1(Sensor_data)
  Error State Kalman Filter/1(delta_state) -> INS propogation/3(delta_state)
  Error State Kalman Filter/2(Measuemrnt Enable Flag) -> INS propogation/2(Measuemrnt Enable Flag)
  INS propogation/1(INSstate) -> Error State Kalman Filter/2(INS state), Bus_Constructor/1(INSstate)
  Bus_Constructor/1(TranslationData) -> TranslationData/1
  Bus_Constructor/2(RotationData) -> RotationData/1
  Sensor_data1/1 -> Error State Kalman Filter/1(Sensor_data)

== system main_RI_LIEKF_GNSSOutrage/State estimation/RI EKF_AOA_ref ==
  Sensor_data : Inport
  Bus_Constructor : Subsystem
  Data Store Memory : DataStoreMemory  DataStoreName=feedback_flag_18dim_RIEKF  WriteAfterWriteMsg=warning  ShowAdditionalParam=off
  Data Store Memory1 : DataStoreMemory  DataStoreName=GPS_enable_RIEKF  WriteAfterWriteMsg=warning  ShowAdditionalParam=off
  Error State Kalman Filter : Subsystem
  INS propogation : Subsystem
  Sensor_data1 : InportShadow
  RotationData : Outport
  TranslationData : Outport  Port=2
  INSbiasData : Outport  Port=3
  EKF_state : Outport  Port=4
  AOA/SA/Wind : Outport  Port=5
  GNSS enable flag : Outport  Port=6
  wires:
  Bus_Constructor/5(GNSS enable flag) -> GNSS enable flag/1
  Bus_Constructor/4(AOA/SA/Wind) -> AOA/SA/Wind/1
  Bus_Constructor/3(INSbiasData) -> INSbiasData/1
  Error State Kalman Filter/3(EKFstate) -> EKF_state/1
  Sensor_data/1 -> INS propogation/1(Sensor_data)
  Error State Kalman Filter/1(delta_state) -> INS propogation/3(delta_state)
  Error State Kalman Filter/2(Measuemrnt Enable Flag) -> INS propogation/2(Measuemrnt Enable Flag)
  INS propogation/1(INSstate) -> Bus_Constructor/1(INSstate), Error State Kalman Filter/2(INS state)
  Bus_Constructor/1(TranslationData) -> TranslationData/1
  Bus_Constructor/2(RotationData) -> RotationData/1
  Sensor_data1/1 -> Error State Kalman Filter/1(Sensor_data)

== system main_RI_LIEKF_GNSSOutrage/State estimation/RI UKF ==
  Sensor_data : Inport
  Bus_Constructor : Subsystem
  Data Store Memory : DataStoreMemory  DataStoreName=feedback_flag_18dim  WriteAfterWriteMsg=warning  ShowAdditionalParam=off
  Data Store Memory1 : DataStoreMemory  DataStoreName=GPS_enable  WriteAfterWriteMsg=warning  ShowAdditionalParam=off
  Data Store Read : DataStoreRead  DataStoreName=GPS_enable  IndexOptions=Index vector (dialog)  Indices=1  OutputSizes=1
  Error State Kalman Filter : Subsystem
  INS propogation : Subsystem
  Scope : Scope
  Sensor_data1 : InportShadow
  TranslationData : Outport
  RotationData : Outport  Port=2
  delta_state : Outport  Port=3
  wires:
  Sensor_data1/1 -> Error State Kalman Filter/1(Sensor_data)
  Error State Kalman Filter/3(covariance) -> Scope/1
  Bus_Constructor/2(RotationData) -> RotationData/1
  Bus_Constructor/1(TranslationData) -> TranslationData/1
  INS propogation/1(INSstate) -> Bus_Constructor/1(INSstate), Error State Kalman Filter/2(INS state)
  Error State Kalman Filter/2(Measuemrnt Enable Flag) -> INS propogation/2(Measuemrnt Enable Flag)
  Error State Kalman Filter/1(delta_state) -> INS propogation/3(delta_state), delta_state/1
  Sensor_data/1 -> INS propogation/1(Sensor_data)

== system main_RI_LIEKF_GNSSOutrage/State estimation/bak1 ==
  Sensor_data : Inport
  Bus_Constructor : Subsystem
  Data Store Memory : DataStoreMemory  DataStoreName=feedback_flag_18dim  WriteAfterWriteMsg=warning  ShowAdditionalParam=off
  Data Store Memory1 : DataStoreMemory  DataStoreName=GPS_enable  WriteAfterWriteMsg=warning  ShowAdditionalParam=off
  Data Store Read : DataStoreRead  DataStoreName=GPS_enable  IndexOptions=Index vector (dialog)  Indices=1  OutputSizes=1
  Error State Kalman Filter : Subsystem
  INS propogation : Subsystem
  Scope : Scope
  Sensor_data1 : InportShadow
  TranslationData : Outport
  RotationData : Outport  Port=2
  delta_state : Outport  Port=3
  wires:
  Sensor_data/1 -> INS propogation/1(Sensor_data)
  Error State Kalman Filter/1(delta_state) -> delta_state/1, INS propogation/3(delta_state)
  Error State Kalman Filter/2(Measuemrnt Enable Flag) -> INS propogation/2(Measuemrnt Enable Flag)
  INS propogation/1(INSstate) -> Error State Kalman Filter/2(INS state), Bus_Constructor/1(INSstate)
  Bus_Constructor/1(TranslationData) -> TranslationData/1
  Bus_Constructor/2(RotationData) -> RotationData/1
  Error State Kalman Filter/3(covariance) -> Scope/1
  Sensor_data1/1 -> Error State Kalman Filter/1(Sensor_data)

== system main_RI_LIEKF_GNSSOutrage/State estimation/distribute CF ==
  Sensor_data : Inport
  AHRS : Subsystem  Commented=on
  Bus Selector : BusSelector  Commented=on  OutputSignals=QGC_sensor_reinit,IMU_Data.accl_B_m/s2_LPF,MAGN_Data,GPS_Data
  Translation_estimate : Subsystem  Commented=on
  distribute CF : Subsystem  mask{att_correct_gain=0.1, att_heading_correct_gain=0.01, gbias_correct_gain=0.1, MAG_GAIN=-0.2}
      mask DialogControl ParameterGroupVar Prompt: 参数
  RotationData : Outport
  TranslationData : Outport  Port=2
  wires:
  AHRS/1(RotationData) -> Translation_estimate/1(RotationData)  "RotationData"
  Bus Selector/2 -> AHRS/2(<accl_B_m/s2_LPF>)  "<accl_B_m/s2_LPF>"
  Bus Selector/3 -> AHRS/3(<MAGN_Data>)  "<MAGN_Data>"
  Bus Selector/1 -> AHRS/1(<QGC_sensor_reinit>)  "<QGC_sensor_reinit>"
  Bus Selector/4 -> AHRS/4(<GPS_Data>)  "<GPS_Data>"
  Sensor_data/1 -> distribute CF/1(Sensor_data), Translation_estimate/2(Sensor_data), AHRS/5(Sensor_data), Bus Selector/1
  distribute CF/1(RotationData) -> RotationData/1
  distribute CF/2(TranslationData) -> TranslationData/1

== system main_RI_LIEKF_GNSSOutrage/Subsystem/Subsystem1 ==
  vel_NED : Inport
  Compare To Constant : simulink/Logic and Bit Operations/Compare To Constant  relop=>=  const=10  OutDataTypeStr=boolean
  Math Function : Math  Operator=magnitude^2
  Sqrt : Sqrt
  Sum of Elements : Sum  Inputs=+
  AOA_Estimation_flag : Outport
  wires:
  Sum of Elements/1 -> Sqrt/1
  Sqrt/1 -> Compare To Constant/1
  Compare To Constant/1 -> AOA_Estimation_flag/1
  Math Function/1 -> Sum of Elements/1
  vel_NED/1 -> Math Function/1

== system main_RI_LIEKF_GNSSOutrage/Subsystem/Subsystem3 ==
  RIEKF_att_Deg : Inport
  vel_NED : Inport  Port=2
  psi_Deg : Inport  Port=3
  Enable : EnablePort
  Add1 : Sum  Inputs=+-
  Add2 : Sum  Inputs=+-
  Asin1 : Trigonometry  Operator=asin
  Atan2 : Trigonometry  Operator=atan2
  Divide1 : Product  Inputs=*/
  Fcn : Fcn  Expr=sqrt(u(1)^2+u(2)^2+u(3)^2)
  Gain : Gain  Gain=-1
  Radians to Degrees1 : simulink_extras/Transformations/Radians to Degrees
  Radians to Degrees3 : simulink_extras/Transformations/Radians to Degrees
  Selector1 : Selector  InputPortWidth=3  IndexOptions=Index vector (dialog)  Indices=[2]  OutputSizes=1
  Selector2 : Selector  InputPortWidth=3  IndexOptions=Index vector (dialog)  Indices=[3]  OutputSizes=1
  Selector3 : Selector  InputPortWidth=3  IndexOptions=Index vector (dialog)  Indices=[1]  OutputSizes=1
  AOA_direct_Deg : Outport
  SA_direct_Deg : Outport  Port=2
  wires:
  RIEKF_att_Deg/1 -> Add1/1
  Radians to Degrees3/1 -> Add1/2  "theta"
  Divide1/1 -> Asin1/1
  Selector2/1 -> Gain/1
  vel_NED/1 -> Selector3/1, Selector1/1, Fcn/1, Selector2/1
  Asin1/1 -> Radians to Degrees3/1
  Fcn/1 -> Divide1/2
  Gain/1 -> Divide1/1
  Add1/1 -> AOA_direct_Deg/1  "AOA_direct"
  Selector1/1 -> Atan2/1
  Selector3/1 -> Atan2/2
  Atan2/1 -> Radians to Degrees1/1
  psi_Deg/1 -> Add2/1
  Radians to Degrees1/1 -> Add2/2  "theta"
  Add2/1 -> SA_direct_Deg/1  "SA_direct"

== system main_RI_LIEKF_GNSSOutrage/Sensor_Data_Process/GPS_Data_Process/LLA2NED ==
  note: Vecef2ned
  gps_LLA_rad : Inport
  GPSfixtype : Inport  Port=2
  GPS_Vecef_m/s : Inport  Port=3
  QGC_sensor_reinit : Inport  Port=4
  Angle Conversion1 : aerolibconvert2/Angle Conversion  IU=deg  OU=rad
  Bus Creator : BusCreator  Inputs=3
  Bus Creator1 : BusCreator  Inputs=3
  Bus Selector : BusSelector  OutputSignals=lon_gps,lat_gps
  Bus Selector1 : BusSelector  OutputSignals=lat_gps,lon_gps,H_gps
  Constant1 : Constant  Value=-90
  Constant4 : Constant  Value=0
  Data Type Conversion{,1..3} (4 alike) : DataTypeConversion  OutDataTypeStr=single  SaturateOnIntegerOverflow=off  RndMeth=Floor
  Demux : Demux  Outputs=3
  Demux1 : Demux  Outputs=3
  Demux3 : Demux  Outputs=3
  Detect Increase : simulink/Logic and Bit Operations/Detect Increase  vinit=0.0  OutDataTypeStr=boolean
  Direction Cosine Matrix ECEF to NED : aerolibtransform2/Direction Cosine Matrix ECEF to NED  Commented=on
  Divide1 : Product  Inputs=**  Multiplication=Matrix(*)
  Gain : Gain  Gain=-1
  LLA to ECEF Position : LLA2ECEF  R=6378137
  LLA to ECEF Position1 : LLA2ECEF  R=6378137
  Mux2 : Mux  Inputs=3
  Mux5 : Mux  Inputs=2
  Mux6 : Mux  Inputs=2
  Product : Product  Commented=on  Multiplication=Matrix(*)
  Radians to Degrees{,1..3} (4 alike) : simulink_extras/Transformations/Radians to Degrees
  Radians to Degrees4 : simulink_extras/Transformations/Radians to Degrees  Commented=on
  Rotation Angles to Direction Cosine Matrix : sharedtransform/Rotation Angles to Direction Cosine Matrix  rotationOrder=ZYX  aMode=aMode
  Scope : Scope  NumInputPorts=2
  Scope1 : Scope
  Selector2 : Selector  Commented=on  InputPortWidth=3  IndexOptions=Index vector (dialog)  Indices=[1 2]  OutputSizes=1
  Sum : Sum  Inputs=|++
  Sum1 : Sum  Inputs=|+-
  initGPSLLA : MATLAB Function  TreatAsAtomicUnit=on
  "gpsposNEDout " : Outport
  gpsvNEDout : Outport  Port=2
  wires:
  initGPSLLA/2(init_GPSLLAflag) -> Scope/1
  initGPSLLA/1(gpsLLA0_rad) -> Scope/2, Demux/1
  Detect Increase/1 -> initGPSLLA/1(QGCinitflag)
  Data Type Conversion3/1 -> gpsvNEDout/1  "gpspos_N"
  Radians to Degrees4/1 -> Direction Cosine Matrix ECEF to NED/1
  Selector2/1 -> Radians to Degrees4/1
  Direction Cosine Matrix ECEF to NED/1 -> Product/1
  GPS_Vecef_m/s/1 -> Product/2, Data Type Conversion3/1
  Radians to Degrees3/1 -> Mux5/2
  Radians to Degrees2/1 -> Mux5/1
  Angle Conversion1/1 -> Sum/2
  Data Type Conversion2/1 -> Bus Creator1/3  "gpspos_D"
  Data Type Conversion1/1 -> Bus Creator1/2  "gpspos_E"
  Data Type Conversion/1 -> Bus Creator1/1  "gpspos_N"
  QGC_sensor_reinit/1 -> Detect Increase/1
  Radians to Degrees1/1 -> Mux6/2
  Radians to Degrees/1 -> Mux6/1
  gps_LLA_rad/1 -> Demux1/1, Selector2/1, initGPSLLA/3(gps_LLA_rad)
  Bus Selector1/3 -> LLA to ECEF Position/2  "<H_gps>"
  Bus Selector1/2 -> Radians to Degrees3/1  "<lon_gps>"
  Bus Selector1/1 -> Radians to Degrees2/1  "<lat_gps>"
  Bus Selector/1 -> Mux2/1  "<lon_gps>"
  Bus Selector/2 -> Gain/1  "<lat_gps>"
  Sum/1 -> Mux2/2
  Demux1/2 -> Radians to Degrees1/1
  LLA to ECEF Position/1 -> Sum1/2
  Constant1/1 -> Angle Conversion1/1
  Rotation Angles to Direction Cosine Matrix/1 -> Divide1/1
  Mux2/1 -> Rotation Angles to Direction Cosine Matrix/1
  Demux1/1 -> Radians to Degrees/1
  Divide1/1 -> Demux3/1
  Sum1/1 -> Divide1/2
  Constant4/1 -> Mux2/3
  LLA to ECEF Position1/1 -> Sum1/1
  Gain/1 -> Sum/1
  Mux5/1 -> LLA to ECEF Position/1
  Mux6/1 -> LLA to ECEF Position1/1
  Demux1/3 -> LLA to ECEF Position1/2
  Demux/1 -> Bus Creator/1  "lat_gps"
  Demux/2 -> Bus Creator/2  "lon_gps"
  Demux/3 -> Bus Creator/3  "H_gps"
  Bus Creator/1 -> Bus Selector1/1, Bus Selector/1
  Demux3/1 -> Data Type Conversion/1  "gpspos_N"
  Demux3/2 -> Data Type Conversion1/1  "gpspos_E"
  Demux3/3 -> Data Type Conversion2/1  "gpspos_D"
  Bus Creator1/1 -> Scope1/1, "gpsposNEDout "/1
  GPSfixtype/1 -> initGPSLLA/2(GPSfixtype)

== system main_RI_LIEKF_GNSSOutrage/Sensor_Data_Process/GPS_Data_Process/heading_GPS ==
  Vned : Inport
  Atan2 : Trigonometry  Operator=atan2
  Compare To Constant : simulink/Logic and Bit Operations/Compare To Constant  relop=>=  const=0.8  OutDataTypeStr=boolean
  Math Function : Math  Operator=magnitude^2  SignedPower=on
  Moving Average1 : dspstat3/Moving Average  Commented=on  Method=Sliding window  ForgettingFactorPort=off  SpecifyWindowLength=on  WindowLength=10  OverlapLength=9  AllowArbitraryInputLength=off  ForgettingFactor=0.9  SimulateUsing=Code generation
  Rate Transition : RateTransition  OutPortSampleTime=GPSdt
  Scope : Scope  NumInputPorts=2
  Scope1 : Scope
  Selector2 : Selector  InputPortWidth=3  IndexOptions=Index vector (dialog)  Indices=[2]  OutputSizes=1
  Selector3 : Selector  InputPortWidth=3  IndexOptions=Index vector (dialog)  Indices=[1]  OutputSizes=1
  Selector4 : Selector  InputPortWidth=3  IndexOptions=Index vector (dialog)  Indices=[1 2]  OutputSizes=1
  Sqrt : Sqrt
  Sum of Elements : Sum  Inputs=+
  heading_GPS_rad : Outport
  heading_GPS_valid : Outport  Port=2
  wires:
  Atan2/1 -> Rate Transition/1
  Rate Transition/1 -> heading_GPS_rad/1, Scope/2, Scope/1
  Compare To Constant/1 -> heading_GPS_valid/1, Scope1/1
  Sqrt/1 -> Compare To Constant/1
  Selector4/1 -> Math Function/1
  Sum of Elements/1 -> Sqrt/1
  Selector3/1 -> Atan2/2
  Vned/1 -> Selector3/1, Selector4/1, Selector2/1
  Math Function/1 -> Sum of Elements/1
  Selector2/1 -> Atan2/1
